simulink model "simulation"  (R2014a)
settings: Solver=ode45  StartTime=0.0  StopTime=10.0  RelTol=1e-3
settings Model: Creator=flp  LastModifiedBy=flp

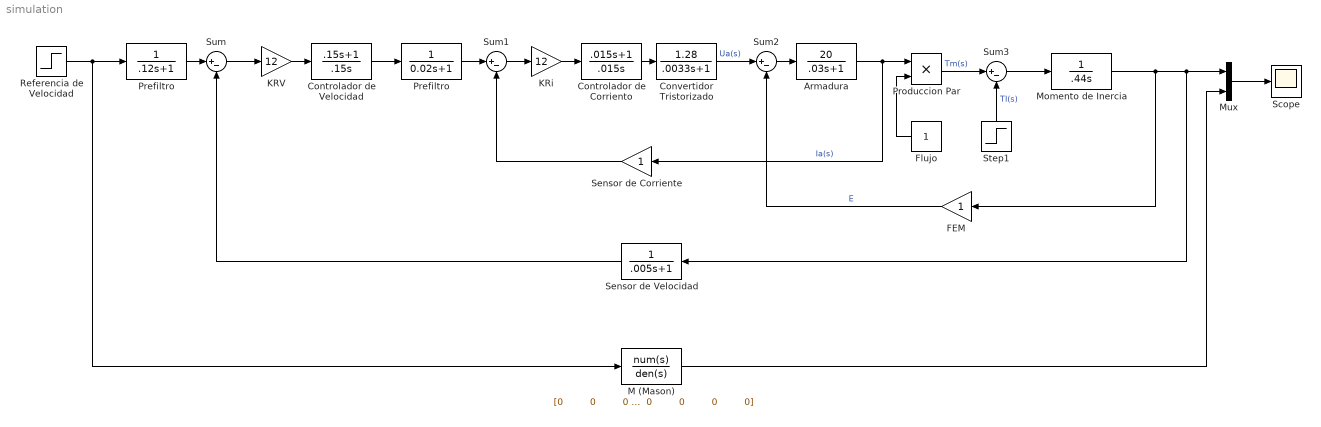
== system simulation ==
  Armadura : TransferFcn  Numerator=[20]  Denominator=[.03 1]
  "Controlador de Corriento " : TransferFcn  Numerator=[.015 1]  Denominator=[.015 0]
  Controlador de Velocidad : TransferFcn  Numerator=[.15 1]  Denominator=[.15 0]
  "Convertidor Tristorizado " : TransferFcn  Numerator=[1.28]  Denominator=[.0033 1]
  FEM : Gain
  Flujo : Constant
  KRV : Gain  Gain=12
  KRi : Gain  Gain=12
  M (Mason) : TransferFcn  Numerator="[0         0         0    0.0000    0.0000    0.0000    0.0000    0.0000    0.0000    0.0000    0.0007 0.0069    0.0241         0         0         0         0         0]"  Denominator="[0.0001   0.0016 0.0097   0.0241         0         0         0         0         0]"
  Momento de Inercia : TransferFcn  Denominator=[.44 0]
  Mux : Mux  Inputs=2
  Prefiltro : TransferFcn  Denominator=[0.02 1]
  "Prefiltro " : TransferFcn  Denominator=[.12 1]
  Produccion Par : Product
  Referencia de Velocidad : Step  Time=0  SampleTime=0
  Scope : Scope
  Sensor de Corriente : Gain
  Sensor de Velocidad : TransferFcn  Denominator=[.005 1]
  Step1 : Step  Time=5  SampleTime=0
  Sum{,1..3} (4 alike) : Sum  Inputs=|+-
  wires:
  Referencia de Velocidad/1 -> M (Mason)/1, "Prefiltro "/1
  "Prefiltro "/1 -> Sum/1
  Sum/1 -> KRV/1
  KRV/1 -> Controlador de Velocidad/1
  Controlador de Velocidad/1 -> Prefiltro/1
  Prefiltro/1 -> Sum1/1
  Sum1/1 -> KRi/1
  KRi/1 -> "Controlador de Corriento "/1
  "Controlador de Corriento "/1 -> "Convertidor Tristorizado "/1
  "Convertidor Tristorizado "/1 -> Sum2/1  "Ua(s)"
  Sum2/1 -> Armadura/1
  Sensor de Velocidad/1 -> Sum/2
  Armadura/1 -> Sensor de Corriente/1, Produccion Par/1  "Ia(s)"
  Produccion Par/1 -> Sum3/1  "Tm(s)"
  Flujo/1 -> Produccion Par/2
  Step1/1 -> Sum3/2  "TI(s)"
  Sum3/1 -> Momento de Inercia/1
  Momento de Inercia/1 -> FEM/1, Sensor de Velocidad/1, Mux/1
  FEM/1 -> Sum2/2  "E"
  Sensor de Corriente/1 -> Sum1/2
  Mux/1 -> Scope/1
  M (Mason)/1 -> Mux/2
